simulink model "integ"  (R2020a)
settings: Solver=VariableStepAuto  StartTime=0.0  StopTime=10.0  RelTol=1e-3
settings Model: Creator=Riyansh  LastModifiedBy=Riyansh

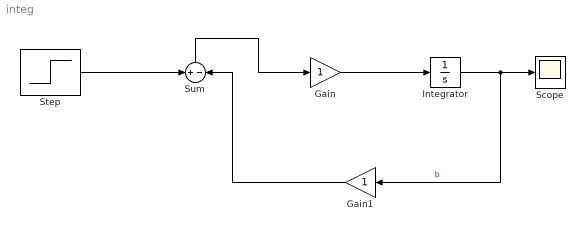
== system integ ==
  Gain : Gain
  Gain1 : Gain
  Integrator : Integrator
  Scope : Scope
  Step : Step  SampleTime=0
  Sum : Sum  Inputs=+-
  wires:
  Gain/1 -> Integrator/1
  Step/1 -> Sum/1
  Sum/1 -> Gain/1
  Integrator/1 -> Gain1/1, Scope/1  "b"
  Gain1/1 -> Sum/2
